simulink model "AC-DC_Rectifier(ZC)"  (R2020a)
settings: Solver=ode23tb  StartTime=0.0  StopTime=0.1  MaxStep=1e-4  RelTol=1e-3  EnableMultiTasking=on
libraries: powerlib x11, dspswit3 x1
settings Model: Creator=Amr Saleh  LastModifiedBy=eslam
settings DataIOCC: LimitDataPoints=on  SaveFormat=Array  ReturnWorkspaceOutputs=off
settings OptimizationCC: LifeSpan=inf
settings DebuggingCC: SolverPrmCheckMsg=warning  SFUnexpectedBacktrackingDiag=warning  SFNoUnconditionalDefaultTransitionDiag=warning  SFExecutionAtInitializationDiag=none  ArithmeticOperatorsInVariantConditions=warning
settings HardwareCC: ProdBitPerPointer=32  ProdBitPerSizeT=32  ProdBitPerPtrDiffT=32  ProdLargestAtomicFloat=None  ProdIntDivRoundTo=Undefined  ProdEndianess=Unspecified  ProdWordSize=32  ProdHWDeviceType=32-bit Generic
settings ModelReferenceCC: PropagateSignalLabelsOutOfModel=off
settings SFSimCC: SimUseLocalCustomCode=off  CustomCodeUndefinedFunction=UseInterfaceOnly
settings RTWCC: RTWUseLocalCustomCode=off
settings CodeAppCC: StateflowObjectComments=on
settings GRTTargetCC: TargetLangStandard=C89/C90 (ANSI)
settings ConfigComp: CovMetricSettings=dw  CovHtmlReporting=on  CovSaveCumulativeToWorkspaceVar=on  CovSaveSingleToWorkspaceVar=on  CovExternalEMLEnable=off  CovSFcnEnable=off
settings SimscapeCC: SimscapeNormalizeSystem=off

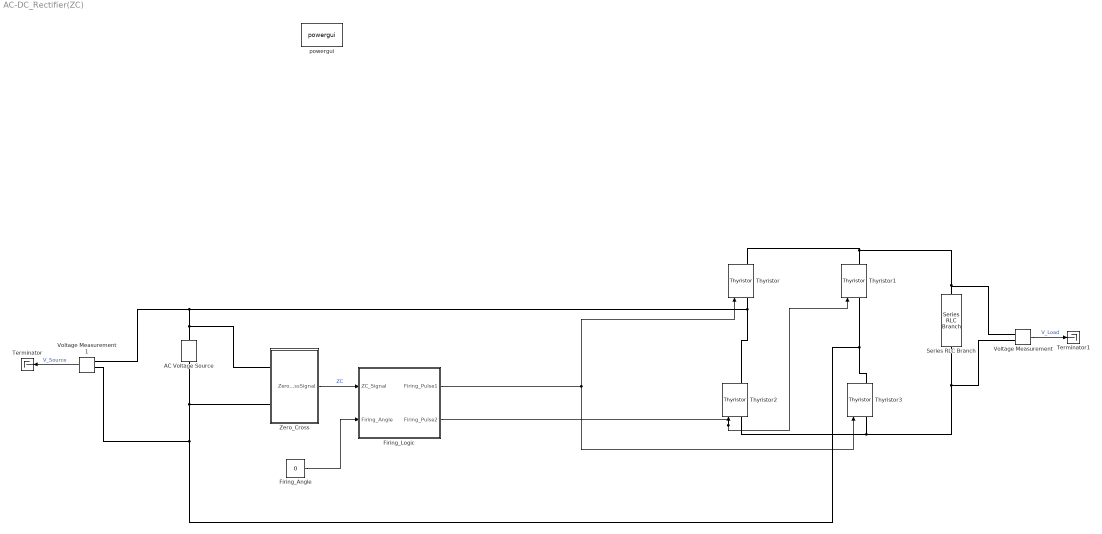
== system AC-DC_Rectifier(ZC) ==
  AC Voltage Source : powerlib/Electrical Sources/AC Voltage Source  Amplitude=240  Phase=0  Frequency=50  SampleTime=0  Measurements=Voltage  BusType=swing  Pref=10e3  Qref=0  Qmin=-inf  Qmax=+inf
  Firing_Angle : Constant  Value=0
  Firing_Logic : Subsystem
  Series RLC Branch : powerlib/Elements/Series RLC Branch  LConnTagsString=__new0  RConnTagsString=__new0  BranchType=R  Resistance=10  Inductance=30e-3  SetiL0=off  InitialCurrent=0  Capacitance=1e-6  Setx0=off  InitialVoltage=0  Measurements=None
  Terminator : Terminator
  Terminator1 : Terminator
  Thyristor{,1..3} (4 alike) : powerlib/Power Electronics/Thyristor  Ron=0.001  Lon=0  Vf=0.8  IC=0  Rs=100  Cs=250e-9  Measurements=on
  Voltage Measurement : powerlib/Measurements/Voltage Measurement  PhasorSimulation=off  OutputType=Complex  PSBequivalent=0
  Voltage Measurement1 : powerlib/Measurements/Voltage Measurement  PhasorSimulation=off  OutputType=Complex  PSBequivalent=0
  Zero_Cross : Subsystem
  powergui : powerlib/powergui  Priority=1  SimulationMode=Continuous  SampleTime=50e-6  frequency=60  Iterations=50  frequencyindice=0  Pbase=100e6  ErrMax=1e-4  UnitsV=kV  UnitsW=MW  buscounter=0  FunctionMessages=off  echomessages=off  EnableUseOfTLC=off  CurrentSourceSwitches=on  DisableSnubberDevices=off  DisableRonSwitches=off  DisableVfSwitches=off  DisplayEquations=off  AutomaticDiscreteSolvers=off  SolverType=Tustin/Backward Euler (TBE)  Interpol=off  ExternalGateDelay=off  methode=off  Ts=100  x0status=blocks  SPID=off  SwTol=0  HookPort=off  NonlinearTolerance=1e-4  nMaxIteration=100  ContinueOnMaxIteration=off  RestoreLinks=warning  ResistiveCurrentMeasurement=off  Frange=[0:2:500]  Ylog=off  Xlog=on  ShowGrid=off  save=off  variable=ZData  structure=0  ZoomFFT=off  StartTime=0.0  cycles=1  DisplayStyle=1  fundamental=60  FreqAxis=off  MaxFrequency=1000  frequencyindicesteady=1  RmsSteady=1  display=off
  wires:
  Voltage Measurement/1 -> Terminator1/1  "V_Load"
  Firing_Angle/1 -> Firing_Logic/2(Firing_Angle)
  Zero_Cross/1(Zero_CrossSignal) -> Firing_Logic/1(ZC_Signal)  "ZC"
  Firing_Logic/1(Firing_Pulse1) -> Thyristor3/1, Thyristor/1
  Firing_Logic/2(Firing_Pulse2) -> Thyristor1/1, Thyristor2/1
  Voltage Measurement1/1 -> Terminator/1  "V_Source"
  connections:
  Voltage Measurement/LConn1 -- Thyristor1/RConn1 -- Thyristor/RConn1 -- Series RLC Branch/LConn1
  AC Voltage Source/RConn1 -- Zero_Cross/LConn2 -- Thyristor3/RConn1 -- Thyristor1/LConn1 -- Voltage Measurement1/LConn1
  Series RLC Branch/RConn1 -- Thyristor2/LConn1 -- Thyristor3/LConn1 -- Voltage Measurement/LConn2
  Voltage Measurement1/LConn2 -- Zero_Cross/LConn1 -- AC Voltage Source/LConn1 -- Thyristor2/RConn1 -- Thyristor/LConn1

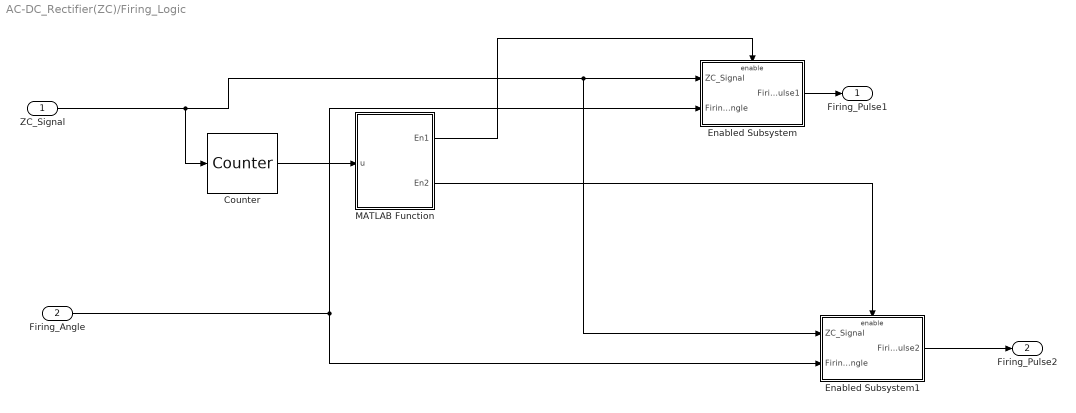
== system AC-DC_Rectifier(ZC)/Firing_Logic ==
  ZC_Signal : Inport
  Firing_Angle : Inport  Port=2
  Counter : dspswit3/Counter  Direction=Up  CountEvent=Rising edge  CounterSize=User defined  MaxCount=255  InitialCount=0  Output=Count  HitValue=32  ResetInput=off  SamplesPerFrame=1  Ts=1  CntDtype=double  HitDtype=Logical
  Enabled Subsystem : Subsystem  TreatAsAtomicUnit=on
  Enabled Subsystem1 : Subsystem  TreatAsAtomicUnit=on
  MATLAB Function : MATLAB Function  TreatAsAtomicUnit=on
  Firing_Pulse1 : Outport
  Firing_Pulse2 : Outport  Port=2
  wires:
  Counter/1 -> MATLAB Function/1(u)
  MATLAB Function/1(En1) -> Enabled Subsystem/Enable
  MATLAB Function/2(En2) -> Enabled Subsystem1/Enable
  ZC_Signal/1 -> Counter/1, Enabled Subsystem1/1(ZC_Signal), Enabled Subsystem/1(ZC_Signal)
  Firing_Angle/1 -> Enabled Subsystem1/2(Firing_Angle), Enabled Subsystem/2(Firing_Angle)
  Enabled Subsystem/1(Firing_Pulse1) -> Firing_Pulse1/1
  Enabled Subsystem1/1(Firing_Pulse2) -> Firing_Pulse2/1

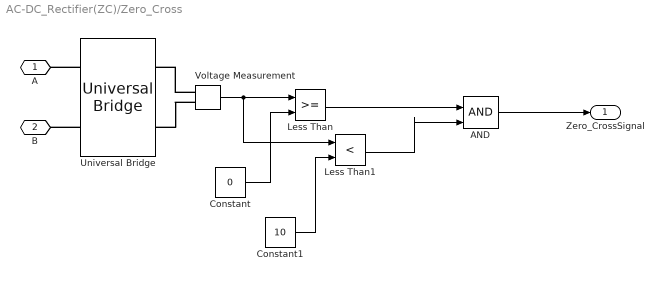
== system AC-DC_Rectifier(ZC)/Zero_Cross ==
  AND : Logic  IconShape=distinctive  AllPortsSameDT=off  OutDataTypeStr=boolean
  Constant : Constant  Value=0
  Constant1 : Constant  Value=10
  Less Than : RelationalOperator  OutDataTypeStr=boolean  RndMeth=Simplest
  Less Than1 : RelationalOperator  Operator=<  OutDataTypeStr=boolean  RndMeth=Simplest
  Universal Bridge : powerlib/Power Electronics/Universal Bridge  Arms=2  SnubberResistance=1e5  SnubberCapacitance=inf  Device=Diodes  Ron=1e-3  Lon=0  ForwardVoltages="[  0  0  ]"  ForwardVoltage=0  GTOparameters=[ 10e-6 , 20e-6 ]  IGBTparameters=[ 1e-6 , 2e-6 ]  Measurements=None  Measurements_2=None  converterType=Rectifier
  Voltage Measurement : powerlib/Measurements/Voltage Measurement  PhasorSimulation=off  OutputType=Complex  PSBequivalent=0
  A : PMIOPort  Side=Left
  B : PMIOPort  Port=2  Side=Left
  Zero_CrossSignal : Outport
  wires:
  Voltage Measurement/1 -> Less Than1/1, Less Than/1
  Constant/1 -> Less Than/2
  Constant1/1 -> Less Than1/2
  Less Than/1 -> AND/1
  Less Than1/1 -> AND/2
  AND/1 -> Zero_CrossSignal/1
  connections:
  Universal Bridge/LConn1 -- A/RConn1
  Universal Bridge/LConn2 -- B/RConn1
  Voltage Measurement/LConn1 -- Universal Bridge/RConn1
  Voltage Measurement/LConn2 -- Universal Bridge/RConn2

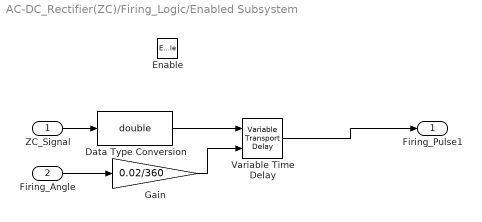
== system AC-DC_Rectifier(ZC)/Firing_Logic/Enabled Subsystem ==
  ZC_Signal : Inport
  Firing_Angle : Inport  Port=2
  Enable : EnablePort
  Data Type Conversion : DataTypeConversion  OutDataTypeStr=double
  Gain : Gain  Gain=0.02/360
  Variable Time Delay : VariableTransportDelay  MaximumDelay=10
  Firing_Pulse1 : Outport
  wires:
  ZC_Signal/1 -> Data Type Conversion/1
  Firing_Angle/1 -> Gain/1
  Data Type Conversion/1 -> Variable Time Delay/1
  Variable Time Delay/1 -> Firing_Pulse1/1
  Gain/1 -> Variable Time Delay/2

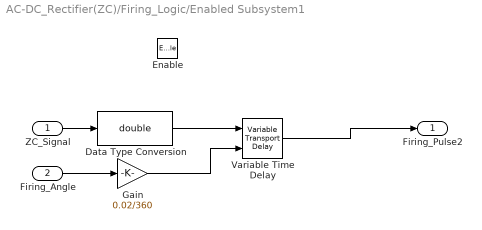
== system AC-DC_Rectifier(ZC)/Firing_Logic/Enabled Subsystem1 ==
  ZC_Signal : Inport
  Firing_Angle : Inport  Port=2
  Enable : EnablePort
  Data Type Conversion : DataTypeConversion  OutDataTypeStr=double
  Gain : Gain  Gain=0.02/360
  Variable Time Delay : VariableTransportDelay  MaximumDelay=10
  Firing_Pulse2 : Outport
  wires:
  ZC_Signal/1 -> Data Type Conversion/1
  Gain/1 -> Variable Time Delay/2
  Data Type Conversion/1 -> Variable Time Delay/1
  Firing_Angle/1 -> Gain/1
  Variable Time Delay/1 -> Firing_Pulse2/1

== matlab function AC-DC_Rectifier(ZC)/Firing_Logic/MATLAB Function ==
  data: u input; En1 output; En2 output
function [En1,En2] = fcn(u)

En1=0;
En2=0;

if mod(u,2)==0
    En1=1;
    En2=0;
end
if mod(u,2)==1
    En1=0;
    En2=1;
end
